simulink model "Rectificador_RL"  (R2023b)
settings: Solver=ode45  StartTime=0.0  StopTime=4  RelTol=1e-3  EnableMultiTasking=on
values from neighbouring files (symbols this model uses):
  L = input('Ingrese el valor de L: ')    [iout.m]    (also in mediaondacontrolado.m = 0.01)
  R = input('Ingrese el valor de R: ')    [iout.m]    (also in mediaondacontrolado.m = 10)
libraries: spsVoltageMeasurementLib x7, spsDiodeLib x6, spsACVoltageSourceLib x3, spsCurrentMeasurementLib x2, spsSeriesRLCBranchLib x2, spsTHDLib x1, sps_lib x1
settings Model: Creator=TGM 612  LastModifiedBy=juanc
settings SolverCC: AlgebraicLoopSolver=TrustRegion
settings DataIOCC: LimitDataPoints=on  SaveFormat=Array  ReturnWorkspaceOutputs=off
settings OptimizationCC: LifeSpan=inf
settings DebuggingCC: FcnCallInpInsideContextMsg=warning  UnconnectedInputMsg=warning  UnconnectedOutputMsg=warning  UnconnectedLineMsg=warning  SFUnexpectedBacktrackingDiag=warning  SFNoUnconditionalDefaultTransitionDiag=warning  SFExecutionAtInitializationDiag=none  ArithmeticOperatorsInVariantConditions=warning
settings HardwareCC: ProdBitPerPointer=32  ProdBitPerSizeT=32  ProdBitPerPtrDiffT=32  ProdLargestAtomicFloat=None  ProdIntDivRoundTo=Undefined  ProdEndianess=Unspecified  ProdWordSize=32  ProdHWDeviceType=32-bit Generic
settings ModelReferenceCC: PropagateSignalLabelsOutOfModel=off
settings SFSimCC: SimUseLocalCustomCode=off  CustomCodeUndefinedFunction=UseInterfaceOnly
settings RTWCC: RTWUseLocalCustomCode=off
settings CodeAppCC: StateflowObjectComments=on
settings GRTTargetCC: TargetLangStandard=C89/C90 (ANSI)
settings ConfigComp: CovMetricSettings=dw  CovSaveCumulativeToWorkspaceVar=on  CovSaveSingleToWorkspaceVar=on  CovExternalEMLEnable=off
settings SimscapeCC: SimscapeNormalizeSystem=off

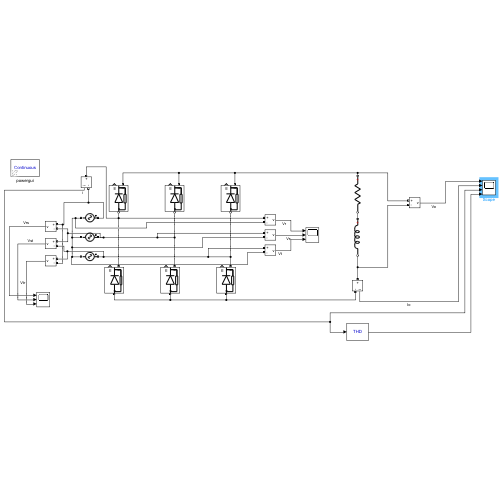
[thumbnail: Simulink's stored preview of the top-level diagram]
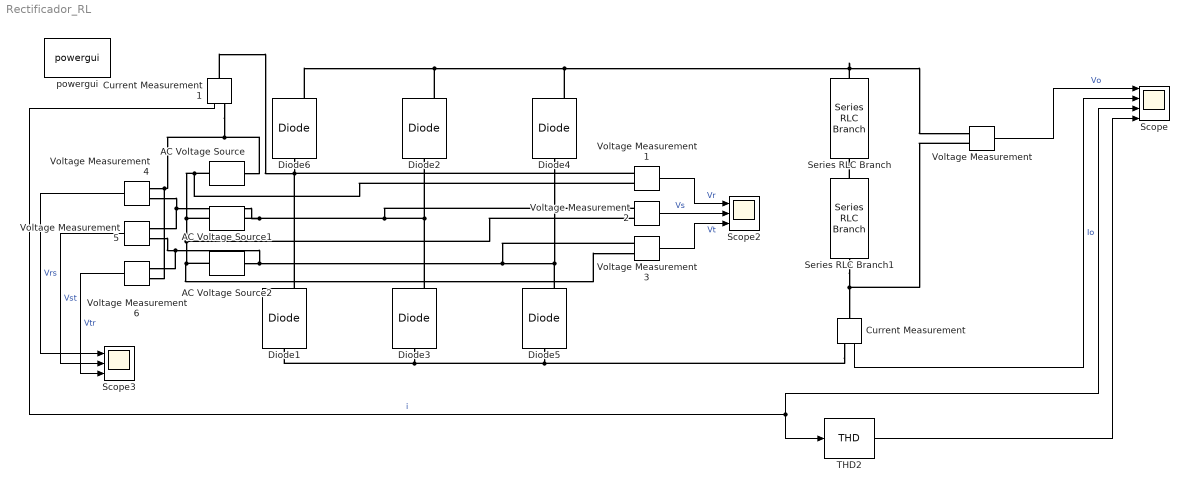
== system Rectificador_RL ==
  AC Voltage Source : spsACVoltageSourceLib/AC Voltage Source  Amplitude=170  Phase=0  Frequency=60  SampleTime=0  Measurements=None  BusType=swing  Pref=10e3  Qref=0  Qmin=-inf  Qmax=+inf
  AC Voltage Source1 : spsACVoltageSourceLib/AC Voltage Source  Amplitude=170  Phase=-120  Frequency=60  SampleTime=0  Measurements=None  BusType=swing  Pref=10e3  Qref=0  Qmin=-inf  Qmax=+inf
  AC Voltage Source2 : spsACVoltageSourceLib/AC Voltage Source  Amplitude=170  Phase=120  Frequency=60  SampleTime=0  Measurements=None  BusType=swing  Pref=10e3  Qref=0  Qmin=-inf  Qmax=+inf
  Current Measurement : spsCurrentMeasurementLib/Current Measurement  PhasorSimulation=off  OutputType=Complex  PSBequivalent=0
  Current Measurement1 : spsCurrentMeasurementLib/Current Measurement  PhasorSimulation=off  OutputType=Complex  PSBequivalent=0
  Diode{1..6} (6 alike) : spsDiodeLib/Diode  Ron=0.001  Lon=0  Vf=0.001  IC=0  UseSnubber=0  Rs=500  Cs=250e-9  Measurements=on
  Scope : Scope  NumInputPorts=4
  Scope2 : Scope  NumInputPorts=3
  Scope3 : Scope  NumInputPorts=3
  Series RLC Branch : spsSeriesRLCBranchLib/Series RLC Branch  LConnTagsString=__new0  RConnTagsString=__new0  BranchType=R  Resistance=R  Inductance=.025  SetiL0=on  InitialCurrent=0  Capacitance=1e-6  Setx0=off  InitialVoltage=0  Measurements=None
  Series RLC Branch1 : spsSeriesRLCBranchLib/Series RLC Branch  LConnTagsString=__new0  RConnTagsString=__new0  BranchType=L  Resistance=10  Inductance=L  SetiL0=on  InitialCurrent=0  Capacitance=1e-6  Setx0=off  InitialVoltage=0  Measurements=None
  THD2 : spsTHDLib/THD  Freq=60  Ts=0
  Voltage Measurement{,1..6} (7 alike) : spsVoltageMeasurementLib/Voltage Measurement  PhasorSimulation=off  OutputType=Complex  PSBequivalent=0
  powergui : sps_lib/powergui  Priority=1  SimulationMode=Continuous  SampleTime=50e-6  frequency=60  Iterations=50  frequencyindice=60  Pbase=100e6  ErrMax=1e-4  UnitsV=kV  UnitsW=MW  buscounter=0  FunctionMessages=off  echomessages=off  EnableUseOfTLC=off  CurrentSourceSwitches=off  DisableSnubberDevices=off  DisableRonSwitches=off  DisableVfSwitches=off  DisplayEquations=off  AutomaticDiscreteSolvers=off  SolverType=Tustin/Backward Euler (TBE)  Interpol=off  ExternalGateDelay=off  methode=off  Ts=100  x0status=blocks  SPID=off  SwTol=0  HookPort=off  NonlinearTolerance=1e-4  nMaxIteration=100  ContinueOnMaxIteration=off  RestoreLinks=warning  ResistiveCurrentMeasurement=off  Frange=[0:2:500]  Ylog=off  Xlog=on  ShowGrid=off  save=off  variable=ZData  structure=0  ZoomFFT=off  StartTime=0.0  cycles=1  DisplayStyle=1  fundamental=60  FreqAxis=off  MaxFrequency=1000  frequencyindicesteady=1  RmsSteady=1  display=off
  wires:
  Voltage Measurement/1 -> Scope/1  "Vo"
  Current Measurement/1 -> Scope/2  "Io"
  Voltage Measurement1/1 -> Scope2/1  "Vr"
  Voltage Measurement2/1 -> Scope2/2  "Vs"
  Voltage Measurement3/1 -> Scope2/3  "Vt"
  Voltage Measurement6/1 -> Scope3/3  "Vtr"
  Voltage Measurement5/1 -> Scope3/2  "Vst"
  Voltage Measurement4/1 -> Scope3/1  "Vrs"
  THD2/1 -> Scope/4
  Current Measurement1/1 -> Scope/3, THD2/1  "i"
  connections:
  Voltage Measurement/LConn2 -- Series RLC Branch1/RConn1 -- Current Measurement/LConn1
  Diode2/RConn1 -- Diode6/RConn1 -- Diode4/RConn1 -- Series RLC Branch/LConn1 -- Voltage Measurement/LConn1
  Series RLC Branch1/LConn1 -- Series RLC Branch/RConn1
  Voltage Measurement6/LConn2 -- Current Measurement1/RConn1 -- AC Voltage Source/RConn1 -- Voltage Measurement4/LConn1
  AC Voltage Source2/LConn1 -- Voltage Measurement1/LConn2 -- AC Voltage Source/LConn1 -- AC Voltage Source1/LConn1 -- Voltage Measurement2/LConn2 -- Voltage Measurement3/LConn2
  Diode3/RConn1 -- Diode2/LConn1 -- Voltage Measurement2/LConn1 -- Voltage Measurement5/LConn1 -- Voltage Measurement4/LConn2 -- AC Voltage Source1/RConn1
  Voltage Measurement6/LConn1 -- Voltage Measurement5/LConn2 -- AC Voltage Source2/RConn1 -- Voltage Measurement3/LConn1 -- Diode4/LConn1 -- Diode5/RConn1
  Diode5/LConn1 -- Current Measurement/RConn1 -- Diode3/LConn1 -- Diode1/LConn1
  Voltage Measurement1/LConn1 -- Diode6/LConn1 -- Current Measurement1/LConn1 -- Diode1/RConn1
